simulink model "Counter_With_Reset_"  (R2022b)
settings: Solver=FixedStepAuto  StartTime=0.0  StopTime=40  FixedStep=1e-3  RelTol=1e-3
settings Model: Creator=yasso  LastModifiedBy=yasso

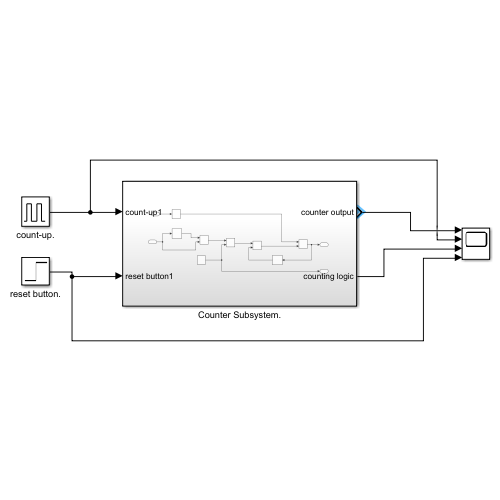
[thumbnail: Simulink's stored preview of the top-level diagram]
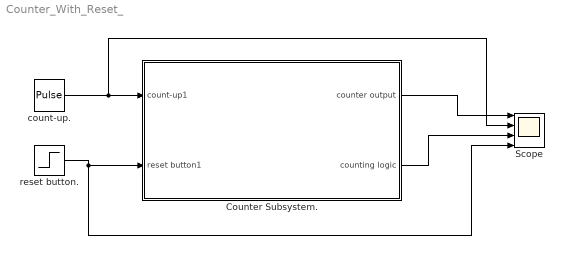
== system Counter_With_Reset_ ==
  Counter Subsystem. : Subsystem
  Scope : Scope  NumInputPorts=4
  count-up. : DiscretePulseGenerator  PulseType=Time based  Period=10  PulseWidth=50  PhaseDelay=5
  reset button. : Step  Time=30  SampleTime=0
  wires:
  count-up./1 -> Scope/2, Counter Subsystem./1(count-up1)
  reset button./1 -> Counter Subsystem./2(reset button1), Scope/4
  Counter Subsystem./1(counter output) -> Scope/1
  Counter Subsystem./2(counting logic) -> Scope/3

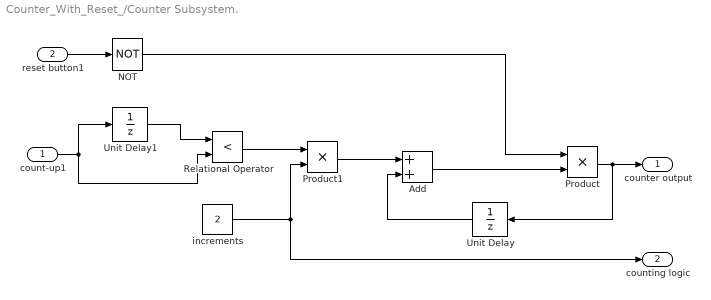
== system Counter_With_Reset_/Counter Subsystem. ==
  count-up1 : Inport
  reset button1 : Inport  Port=2
  Add : Sum
  NOT : Logic  Operator=NOT  AllPortsSameDT=off  OutDataTypeStr=fixdt(1,16)
  Product : Product  OutDataTypeStr=int16
  Product1 : Product
  Relational Operator : RelationalOperator  Operator=<  OutDataTypeStr=boolean  RndMeth=Simplest  InputSameDT=off
  Unit Delay : UnitDelay  SampleTime=-1  HasFrameUpgradeWarning=on
  Unit Delay1 : UnitDelay  SampleTime=-1  HasFrameUpgradeWarning=on
  increments : Constant  Value=2
  counter output : Outport
  counting logic : Outport  Port=2
  wires:
  reset button1/1 -> NOT/1
  Add/1 -> Product/2
  Unit Delay/1 -> Add/2
  Product/1 -> counter output/1, Unit Delay/1
  NOT/1 -> Product/1
  count-up1/1 -> Unit Delay1/1, Relational Operator/2
  Unit Delay1/1 -> Relational Operator/1
  Product1/1 -> Add/1
  Relational Operator/1 -> Product1/1
  increments/1 -> counting logic/1, Product1/2
